simulink model "Msctest2"  (R2017a)
settings: Solver=FixedStepAuto  StartTime=0.0  StopTime=10.0  FixedStep=0.01  RelTol=1e-3
settings Model: Creator=Leonard  LastModifiedBy=ASUS
settings DataIOCC: ReturnWorkspaceOutputs=on
settings SFSimCC: SimUseLocalCustomCode=on
settings RTWCC: RTWUseLocalCustomCode=on

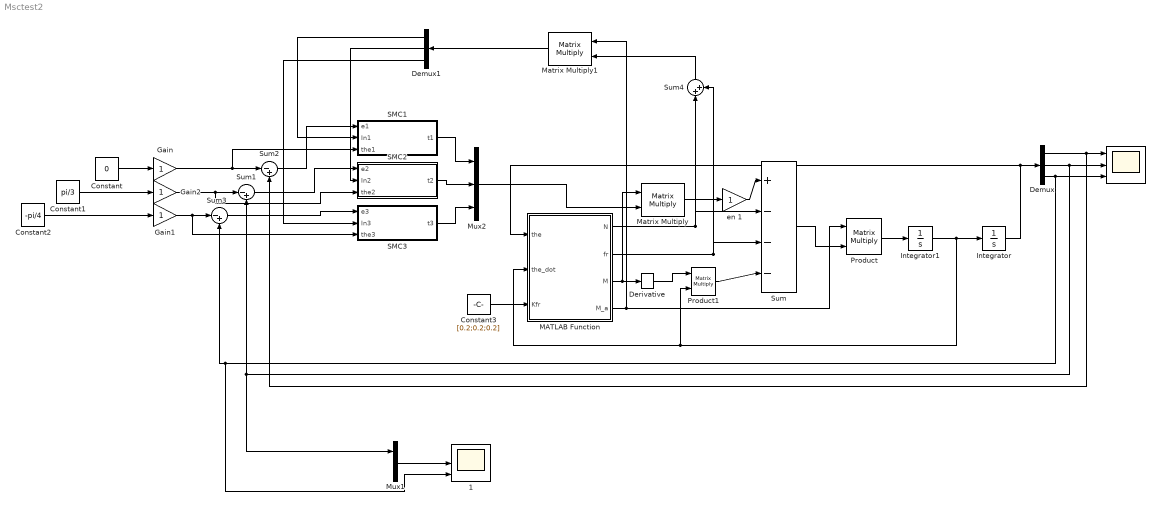
== system Msctest2 ==
  " " : Scope  NumInputPorts=3
  " 1" : Scope  NumInputPorts=3
  Constant : Constant  Value=0
  Constant1 : Constant  Value=pi/3
  Constant2 : Constant  Value=-pi/4
  Constant3 : Constant  Value=[0.2;0.2;0.2]
  Demux : Demux  Outputs=3
  Demux1 : Demux  Outputs=3
  Derivative : Derivative
  Gain : Gain
  Gain1 : Gain
  Gain2 : Gain
  Integrator : Integrator  InitialCondition=[0;0;0]
  Integrator1 : Integrator  InitialCondition=[0;0;0]
  MATLAB Function : MATLAB Function  TreatAsAtomicUnit=on
  Matrix Multiply : Product  Multiplication=Matrix(*)
  Matrix Multiply1 : Product  Multiplication=Matrix(*)
  Mux1 : Mux  Inputs=2
  Mux2 : Mux  Inputs=3
  Product : Product  Multiplication=Matrix(*)
  Product1 : Product  Multiplication=Matrix(*)
  "SMC1 " : Subsystem
  "SMC2 " : Subsystem
  "SMC3 " : Subsystem
  Sum : Sum  Inputs=|+---
  Sum1 : Sum  Inputs=|-+
  Sum2 : Sum  Inputs=|-+
  Sum3 : Sum  Inputs=|-+
  Sum4 : Sum  Inputs=|++
  en 1 : Gain
  wires:
  MATLAB Function/1(N) -> Sum4/1, Sum/2
  Demux/1 -> " "/1, Sum2/2
  Constant3/1 -> MATLAB Function/3(Kfr)
  Demux/2 -> " "/2, Mux1/1, Sum1/2
  Demux/3 -> " "/3, " 1"/3, Sum3/2
  Constant/1 -> Gain/1
  MATLAB Function/3(M) -> Matrix Multiply/1, Derivative/1
  Gain1/1 -> "SMC3 "/3("the3 "), Sum3/1
  Gain/1 -> "SMC1 "/3(the1), Sum2/1
  Integrator/1 -> Demux/1, MATLAB Function/1(the)
  Product/1 -> Integrator1/1
  Derivative/1 -> Product1/1
  Integrator1/1 -> Integrator/1, MATLAB Function/2(the_dot), Product1/2
  MATLAB Function/2(fr) -> Sum/3, Sum4/2
  Product1/1 -> Sum/4
  en 1/1 -> Sum/1
  MATLAB Function/4(M_a) -> Matrix Multiply1/1, Product/1
  Sum/1 -> Product/2
  Gain2/1 -> "SMC2 "/3("the2 "), Sum1/1
  Sum3/1 -> "SMC3 "/1(e3)
  Sum1/1 -> "SMC2 "/1(e2)
  Sum2/1 -> "SMC1 "/1(e1)
  "SMC2 "/1("t2 ") -> Mux2/2
  "SMC1 "/1(t1) -> Mux2/1
  "SMC3 "/1(t3) -> Mux2/3
  Demux1/2 -> "SMC2 "/2(In2)
  Demux1/3 -> "SMC3 "/2(In3)
  Demux1/1 -> "SMC1 "/2(In1)
  Matrix Multiply/1 -> en 1/1
  Mux2/1 -> Matrix Multiply/2
  Mux1/1 -> " 1"/2
  Matrix Multiply1/1 -> Demux1/1
  Sum4/1 -> Matrix Multiply1/2
  Constant1/1 -> Gain2/1
  Constant2/1 -> Gain1/1

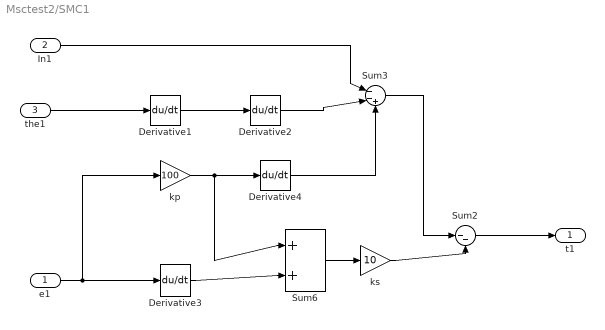
== system Msctest2/SMC1  ==
  e1 : Inport
  In1 : Inport  Port=2
  the1 : Inport  Port=3
  Derivative{1..4} (4 alike) : Derivative
  Sum2 : Sum  Inputs=|--
  Sum3 : Sum  Inputs=|--+
  Sum6 : Sum  Inputs=|++
  kp : Gain  Gain=100
  "ks " : Gain  Gain=10
  t1 : Outport
  wires:
  Derivative1/1 -> Derivative2/1
  Derivative3/1 -> Sum6/2
  Sum6/1 -> "ks "/1
  Sum2/1 -> t1/1
  Sum3/1 -> Sum2/1
  In1/1 -> Sum3/1
  "ks "/1 -> Sum2/2
  Derivative2/1 -> Sum3/2
  kp/1 -> Sum6/1, Derivative4/1
  Derivative4/1 -> Sum3/3
  e1/1 -> kp/1, Derivative3/1
  the1/1 -> Derivative1/1

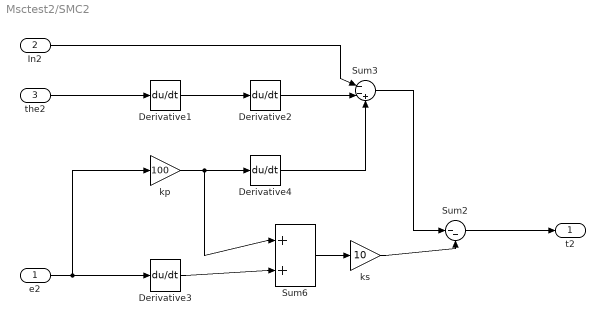
== system Msctest2/SMC2  ==
  e2 : Inport
  In2 : Inport  Port=2
  "the2 " : Inport  Port=3
  Derivative{1..4} (4 alike) : Derivative
  Sum2 : Sum  Inputs=|--
  Sum3 : Sum  Inputs=|--+
  Sum6 : Sum  Inputs=|++
  kp : Gain  Gain=100
  "ks " : Gain  Gain=10
  "t2 " : Outport
  wires:
  Derivative1/1 -> Derivative2/1
  Derivative3/1 -> Sum6/2
  Sum6/1 -> "ks "/1
  Sum2/1 -> "t2 "/1
  Sum3/1 -> Sum2/1
  In2/1 -> Sum3/1
  "ks "/1 -> Sum2/2
  Derivative2/1 -> Sum3/2
  kp/1 -> Sum6/1, Derivative4/1
  Derivative4/1 -> Sum3/3
  e2/1 -> kp/1, Derivative3/1
  "the2 "/1 -> Derivative1/1

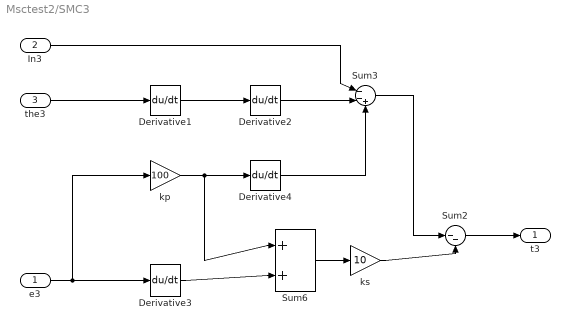
== system Msctest2/SMC3  ==
  e3 : Inport
  In3 : Inport  Port=2
  "the3 " : Inport  Port=3
  Derivative{1..4} (4 alike) : Derivative
  Sum2 : Sum  Inputs=|--
  Sum3 : Sum  Inputs=|--+
  Sum6 : Sum  Inputs=|++
  kp : Gain  Gain=100
  "ks " : Gain  Gain=10
  t3 : Outport
  wires:
  Derivative1/1 -> Derivative2/1
  Derivative3/1 -> Sum6/2
  Sum6/1 -> "ks "/1
  Sum2/1 -> t3/1
  Sum3/1 -> Sum2/1
  In3/1 -> Sum3/1
  "ks "/1 -> Sum2/2
  Derivative2/1 -> Sum3/2
  kp/1 -> Sum6/1, Derivative4/1
  Derivative4/1 -> Sum3/3
  e3/1 -> kp/1, Derivative3/1
  "the3 "/1 -> Derivative1/1

== matlab function Msctest2/MATLAB Function ==
  data: the input; N output; fr output; M output; M_a output; the_dot input; Kfr input
function [N,fr,M,M_a] = fcn(the,the_dot,Kfr)
the1=the(1); the2=the(2); the3=the(3);
L1 = 0.2; L2 = 0.5 ; L3= 0.5; %Link length
m1 = 2 ; m2 = 0.3 ; m3 =0.1 ; %Link mass
%clc
%clear all;
%syms m1 m2 m3 L2 L3 the1 the2 the3 L1 the1_dot the2_dot the3_dot ;
%the_dot = [the1_dot; the2_dot;the3_dot];
%%%%%%%%%%%%%%%%%%%%%%%%%%%%%%%%%%%%%

%TINH JACOBIAN CHO DIEM m1
%P_0_m1 = [ 0; 0; L1];

%DAO HAM P_0_m1 THEO THE1
J_0_m1_dot_the1 = [ 0; 0; 0];
%DAO HAM P_0_m1 THEO THE2
J_0_m1_dot_the2 = [ 0; 0; 0];
%DAO HAM P_0_m1 THEO THE3
J_0_m1_dot_the3 = [ 0; 0; 0]; 

J_0_m1 = [J_0_m1_dot_the1 J_0_m1_dot_the2 J_0_m1_dot_the3];
%%%%%%%%%%%%%%%%%%%%%%%%%%%%%%%%%%%%%%%
%TINH JACOBIAN CHO DIEM m2
%P_0_m2 = [L2*cos(the1)*cos(the2); L2*cos(the2)*sin(the1); L1 + L2*sin(the2)];

%DAO HAM P_0_m2 THEO THE1
J_0_m2_dot_the1 = [L2*sin(-the1)*cos(the2);L2*cos(the2)*cos(the1); 0];
%DAO HAM P_0_m2 THEO THE2
J_0_m2_dot_the2 = [L2*cos(the1)*sin(-the2);L2*sin(-the2)*sin(the1); L2*cos(the2)];
%DAO HAM P_0_m2 THEO THE3
J_0_m2_dot_the3 = [ 0; 0; 0]; 

J_0_m2 = [J_0_m2_dot_the1  J_0_m2_dot_the2  J_0_m2_dot_the3];
%%%%%%%%%%%%%%%%%%%%%%%%%%%%%%%%%%%%%%%%%

%TINH JACOBIAN CHO DIEM m3
%P_0_m3 = [ cos(the1)*(L3*cos(the2 + the3) + L2*cos(the2)); sin(the1)*(L3*cos(the2 + the3) + L2*cos(the2)); L1 + L3*sin(the2 + the3) + L2*sin(the2)];
%DAO HAM P_0_m3 THEO THE1
J_0_m3_dot_the1 = [sin(-the1)*(L3*cos(the2 + the3) + L2*cos(the2));	 cos(the1)*(L3*cos(the2 + the3) + L2*cos(the2));     0];
%DAO HAM P_0_m3 THEO THE2
J_0_m3_dot_the2 = [cos(the1)*(L3*sin(-the2 - the3) + L2*sin(-the2));  sin(the1)*(L3*sin(-the2 - the3) + L2*sin(-the2));    L3*cos(the2 + the3) + L2*cos(the2)];
%DAO HAM P_0_m3 THEO THE3
J_0_m3_dot_the3 = [ cos(the1)*L3*sin(-the2 - the3);	 sin(the1)*L3*sin(-the2 - the3);  L3*cos(the2 + the3)];

J_0_m3 = [J_0_m3_dot_the1  J_0_m3_dot_the2  J_0_m3_dot_the3];

%%%%%%%%%%%%%%%%%%%%%%%%%%%%%%%%%%%%%%%%%%%%%%%%%%%%%%%%%%
%TONG HOP MA TRAN M3

M3 = (m3*[0 0 1]*transpose(J_0_m3)*J_0_m3)

%%%%%%%%%%%%%%%%%%%%%%%%%%%%%%%%%%%%%%%%%%%%%%%%%%%
%TONG HOP MA TRAN M2

M2 = (m2*[0 1 0]*transpose(J_0_m2)*J_0_m2 + m3*[0 1 0]*transpose(J_0_m3)*J_0_m3) 

%%%%%%%%%%%%%%%%%%%%%%%%%%%%%%%%%%%%%%%%%%%%%%%%%%%
%TONG HOP MA TRAN M1

M1 = (m1*[1 0 0]*transpose(J_0_m1)*J_0_m1 + m2*[1 0 0]*transpose(J_0_m2)*J_0_m2 + m3*[1 0 0]*transpose(J_0_m2)*J_0_m3)


M  = [ M1 ; M2 ; M3];
M_a = inv(M);


%%%%%%%%%%%%%%%%%%%%%%%%%%%%%%%%%%%%%%%%%%%%%%%%%%%%%%
 
%DAO HAM J_0_m1_dot_the1 theo the1

J_0_m1_dot_the1_dot_the1 = [ 0; 0; 0];
%DAO HAM J_0_m1_dot_the2 theo the1
J_0_m1_dot_the2_dot_the1 = [ 0; 0; 0];  
%DAO HAM J_0_m1_dot_the3 theo the1
J_0_m1_dot_the3_dot_the1 = [ 0; 0; 0]; 

%DAO HAM J_0_m1 theo the1 
J_0_m1_dot_the1_1 = [J_0_m1_dot_the1_dot_the1  J_0_m1_dot_the2_dot_the1  J_0_m1_dot_the3_dot_the1];

%%%%%%%%%%%%%%%%%%%%%%%%%%%%%%%%%%%%%%%%%%%%%%%%%%%%%%%%%%
%DAO HAM J_0_m2_dot_the1 theo the1
%J_0_m2_dot_the1 = [L2*sin(-the1)*cos(the2);    L2*cos(the2)*cos(the1);  0];
J_0_m2_dot_the1_dot_the1 = [L2*cos(the1)*cos(the2);L2*cos(the2)*sin(-the1); 0];
%DAO HAM J_0_m2_dot_the2 theo the1
%J_0_m2_dot_the2 = [L2*cos(the1)*sin(-the2);    L2*sin(-the2)*sin(the1);     L2*cos(the2)];
J_0_m2_dot_the2_dot_the1 = [L2*sin(the1)*sin(the2);L2*sin(-the2)*cos(the1); 0];
%DAO HAM J_0_m2_dot_the3 theo the1
J_0_m2_dot_the3_dot_the1 = [ 0; 0; 0]; 

%DAO HAM J_0_m2 theo the1 
J_0_m2_dot_the1_1 = [J_0_m2_dot_the1_dot_the1   J_0_m2_dot_the2_dot_the1  J_0_m2_dot_the3_dot_the1];

%%%%%%%%%%%%%%%%%%%%%%%%%%%%%%%%%%%%%%%%%%%%%%%%%%%%%%%%%%%
%DAO HAM J_0_m2_dot_the1 theo the2
%J_0_m2_dot_the1 = [L2*sin(-the1)*cos(the2);    L2*cos(the2)*cos(the1);  0];
J_0_m2_dot_the1_dot_the2 = [L2*sin(the1)*sin(the2);L2*sin(-the2)*cos(the1); 0];
%DAO HAM J_0_m2_dot_the2 theo the2
%J_0_m2_dot_the2 = [L2*cos(the1)*sin(-the2);    L2*sin(-the2)*sin(the1);     L2*cos(the2)];
J_0_m2_dot_the2_dot_the2 = [L2*cos(the1)*cos(the2);L2*cos(the2)*sin(the1); L2*sin(-the2)];
%DAO HAM J_0_m2_dot_the3 theo the2
J_0_m2_dot_the3_dot_the2 = [ 0; 0; 0]; 

%DAO HAM J_0_m2 theo the2
J_0_m2_dot_the2_2 = [J_0_m2_dot_the1_dot_the2  J_0_m2_dot_the2_dot_the2  J_0_m2_dot_the3_dot_the2];

%%%%%%%%%%%%%%%%%%%%%%%%%%%%%%%%%%%%%%%%%%%%%%%%%%%%%%%%%%%%%%%
%DAO HAM J_0_m3_dot_the1 theo the1
%J_0_m3_dot_the1 = [sin(-the1)*(L3*cos(the2 + the3) + L2*cos(the2));	 cos(the1)*(L3*cos(the2 + the3) + L2*cos(the2));     0];
J_0_m3_dot_the1_dot_the1 = [cos(the1)*(L3*cos(the2 + the3) + L2*cos(the2));	 sin(-the1)*(L3*cos(the2 + the3) + L2*cos(the2));     0];
%DAO HAM J_0_m3_dot_the2 theo the1
%J_0_m3_dot_the2 =          [cos(the1)*(L3*sin(-the2 - the3) + L2*sin(-the2));  sin(the1)*(L3*sin(-the2 - the3) + L2*sin(-the2));    L3*cos(the2 + the3) + L2*cos(the2)];
J_0_m3_dot_the2_dot_the1 = [sin(the1)*(L3*sin(the2 + the3) + L2*sin(the2));  -cos(the1)*(L3*sin(the2 + the3) + L2*sin(the2));    0];
%DAO HAM J_0_m3_dot_the3 theo the1
%J_0_m3_dot_the3 =          [ cos(the1)*L3*sin(-the2 - the3);	 sin(the1)*L3*sin(-the2 - the3);  L3*cos(the2 + the3)];
J_0_m3_dot_the3_dot_the1 = [ sin(the1)*L3*sin(the2 + the3);     -cos(the1)*L3*sin(the2 + the3);  0];

J_0_m3_dot_the1_1 = [J_0_m3_dot_the1_dot_the1  J_0_m3_dot_the2_dot_the1  J_0_m3_dot_the3_dot_the1];

%%%%%%%%%%%%%%%%%%%%%%%%%%%%%%%%%%%%%%%%%%%%%%%%%%%%%%%%%%%%%

%DAO HAM J_0_m3_dot_the1 theo the2
%J_0_m3_dot_the1 =          [sin(-the1)*(L3*cos(the2 + the3) + L2*cos(the2));	 cos(the1)*(L3*cos(the2 + the3) + L2*cos(the2));     0];
J_0_m3_dot_the1_dot_the2 = [sin(the1)*(L3*sin(the2 + the3) + L2*sin(the2));	 -cos(the1)*(L3*sin(the2 + the3) + L2*sin(the2));     0];
%DAO HAM J_0_m3_dot_the2 theo the2
%J_0_m3_dot_the2 =        [cos(the1)*(L3*sin(-the2 - the3) + L2*sin(-the2));  sin(the1)*(L3*sin(-the2 - the3) + L2*sin(-the2));    L3*cos(the2 + the3) + L2*cos(the2)];
J_0_m3_dot_the2_dot_the2 = [cos(the1)*(L3*cos(the2 + the3) + L2*cos(the2));  sin(the1)*(L3*cos(the2 + the3) + L2*cos(the2));    -L3*sin(the2 + the3) - L2*sin(the2)];
%DAO HAM J_0_m3_dot_the3 theo the2
%J_0_m3_dot_the3 =         [ cos(the1)*L3*sin(-the2 - the3);	 sin(the1)*L3*sin(-the2 - the3);  L3*cos(the2 + the3)];
J_0_m3_dot_the3_dot_the2 = [ cos(the1)*L3*cos(the2 + the3);     sin(the1)*L3*cos(the2 + the3);  -L3*sin(the2 + the3)];

%DAO HAM J_0_m3 theo the2
J_0_m3_dot_the2_2= [J_0_m3_dot_the1_dot_the2  J_0_m3_dot_the2_dot_the2  J_0_m3_dot_the3_dot_the2];
 

%%%%%%%%%%%%%%%%%%%%%%%%%%%%%%%%%%%%%%%%%%%%%%%%%%%%%%%%%%%%%
%DAO HAM J_0_m3_dot_the1 theo the3
%J_0_m3_dot_the1 =         [sin(-the1)*(L3*cos(the2 + the3) + L2*cos(the2));	 cos(the1)*(L3*cos(the2 + the3) + L2*cos(the2));     0];
J_0_m3_dot_the1_dot_the3 = [sin(the1)*L3*sin(the2 + the3);	 -cos(the1)*L3*sin(the2 + the3);     0];
%DAO HAM J_0_m3_dot_the2 theo the3
%J_0_m3_dot_the2 =        [cos(the1)*(L3*sin(-the2 - the3) + L2*sin(-the2));  sin(the1)*(L3*sin(-the2 - the3) + L2*sin(-the2));    L3*cos(the2 + the3) + L2*cos(the2)];
J_0_m3_dot_the2_dot_the3 = [cos(the1)*L3*cos(the2 + the3);  sin(the1)*L3*cos(the2 + the3);    -L3*sin(the2 + the3)];
%DAO HAM J_0_m3_dot_the3 theo the3
%J_0_m3_dot_the3 =         [ cos(the1)*L3*sin(-the2 - the3);	 sin(the1)*L3*sin(-the2 - the3);  L3*cos(the2 + the3)];
J_0_m3_dot_the3_dot_the3 = [ cos(the1)*L3*cos(the2 + the3);	 sin(the1)*L3*cos(the2 + the3);  -L3*sin(the2 + the3)];

%DAO HAM J_0_m3 theo the3
J_0_m3_dot_the3_3 = [J_0_m3_dot_the1_dot_the3 J_0_m3_dot_the2_dot_the3  J_0_m3_dot_the3_dot_the3];
 
%%%%%%%%%%%%%%%%%%%%%%%%%%%%%%%%%%%%%%%%%%%%%%%%%%%%%%%%%%%%%%%%%
dT_dthe3 = transpose(the_dot)*(m3*transpose(J_0_m3_dot_the3_3)*J_0_m3)*the_dot;
%%%%%%%%%%%%%%%%%%%%%%%%%%%%%%%%%%%%%%%%%%%%
dT_dthe2 = transpose(the_dot)*(m2*transpose(J_0_m2_dot_the2_2)*J_0_m2+m3*transpose(J_0_m3_dot_the2_2)*J_0_m3)*the_dot;
%%%%%%%%%%%%%%%%%%%%%%%%%%%%%%%%%%%%%%%%%%
dT_dthe1 = (transpose(the_dot)*(m1*transpose(J_0_m1_dot_the1_1)*J_0_m1+m2*transpose(J_0_m2_dot_the1_1)*J_0_m2+m3*transpose(J_0_m3_dot_the1_1)*J_0_m3)*the_dot);

%%%%%%%%%%%%%%%%%%%%%%%%%%%%%%%%%%%%%%%%%%%%%%%%%%%%%%%%%%%%%%%%%%
%M3_dot_t = [ 0,	 (L3*m3*L2*sin(-the3))*the3_dot,	 0];
%M2_dot_t = [ 0, (2*L2*L3*m3*sin(-the3))*the3_dot, 	(L3*m3*L2*sin(-the3))*the3_dot];
%M1_dot_t = [ (2*L2^2*m2*cos(the2)*sin(-the2) + 2*L2^2*m3*cos(the2)*sin(-the2) + 2*L2*L3*m3*cos(the2)*sin(-the2)*cos(the3) - L2*L3*m3*sin(-the2)*cos(the2)*sin(the3))*the2_dot + (L2*L3*m3*cos(the2)^2*sin(-the3) - L2*L3*m3*cos(the2)*sin(the2)*cos(the3))*the3_dot,	 0,	0];

%M_dot_t = [ M1_dot_t;M2_dot_t;M3_dot_t];


%%%%%%%%%%%%%%%%%%%%%%%%%%%%%%%%%%%%%%%%%%%%%%%%%%%%%%%%%
%TINH dU_DTHE3
%%%%%%%%%%%%%%%%%%%%%%%%%%%%%%%%%%%%%%%%%%%%%%%%%%%%%%%%%%%%%%%
g_0 = [ 0;0;-9.81];

dU_dthe3 = -m3*transpose(g_0)*J_0_m3_dot_the3
 
N3 = -dT_dthe3 + dU_dthe3;
%V3 = simplify(-dT_dthe3+M3_dot_t*the_dot)
%%%%%%%%%%%%%%%%%%%%%%%%%%%%%%%%%%%%%%%%%%%%%%%%%%%%%%%%%%%
%TINH dU_DTHE2
%%%%%%%%%%%%%%%%%%%%%%%%%%%%%%%%%%%%%%%%%%%%%%%%%%%%%%%%%%%%%%%
g_0 = [ 0;0;-9.81];

dU_dthe2 = -m2*transpose(g_0)*J_0_m2_dot_the2 - m3*transpose(g_0)*J_0_m3_dot_the2
 
N2= -dT_dthe2 + dU_dthe2;
%V2 = simplify(-dT_dthe2 + M2_dot_t*the_dot)
%%%%%%%%%%%%%%%%%%%%%%%%%%%%%%%%%%%%%%%%%%%%%%%%%%%%%%%%%%%
%TINH dU_DTHE1
%%%%%%%%%%%%%%%%%%%%%%%%%%%%%%%%%%%%%%%%%%%%%%%%%%%%%%%%%%%%%%%
g_0 = [ 0;0;-9.81];

dU_dthe1 = -m1*transpose(g_0)*J_0_m1_dot_the1-m2*transpose(g_0)*J_0_m2_dot_the1-m3*transpose(g_0)*J_0_m3_dot_the1
 
N1= -dT_dthe1  + dU_dthe1;
%V1 = simplify(-dT_dthe1+M1_dot_t*the_dot)
N = [ N1;N2;N3] ;
fr = [(Kfr(1)*the_dot(1)); (Kfr(2)*the_dot(2)) ; (Kfr(3)*the_dot(3))];

%%%%%%%%%%%%%%%%%%%%%%%%%%%%%%%%%%%%%%%%%%%%%%%%%%%%%%%%
%PHUONG TRINH DONG LUC HOC
%M*the_2dot + N =to
